simulink library "pmm"  (R2021b)
settings: Solver=VariableStepAuto  StartTime=0.0  StopTime=10.0  RelTol=1e-3
undefined symbols (not defined in the file or in its folder): APMM_CoolgFanActCurr_X_pct, APMM_EWP1Curr_X_c, APMM_EWP3Curr_X_c, APMM_LVBattChktime_X_enum, APMM_LVBattChrgtime_X_enum, APMM_LVChrgLv_X_mV, ENUM_ANTITHEFT_ALARM, ENUM_ANTITHEFT_ARM, ENUM_ANTITHEFT_DISARM, ENUM_ANTITHEFT_WAIT, ENUM_APSSYSTEMSTA_REMOTEACTIVE, ENUM_CHRGPLUGSTA_NONE, ENUM_CRASHSTATE_FRONTFIRSTLV, ENUM_CRASHSTATE_LEFTSIDE, ENUM_CRASHSTATE_RIGHTSIDE, ENUM_DRIVETRAIN_AWD, ENUM_DRIVETRAIN_FWD, ENUM_DRIVETRAIN_RWD, ENUM_GEARACTUALPOSN_D, ENUM_GEARACTUALPOSN_N, ENUM_GEARACTUALPOSN_R, ENUM_HVBATTREADYPRE_READY, ENUM_OTACHKSTA_NOREQUEST, ENUM_OTACHKSTA_NOTIMEOUT, ENUM_OTACHKSTA_TIMEOUT, ENUM_PDKEYRAWLULOCK_INLOCK, ENUM_PDKEYRAWLULOCK_INUNLOCK, ENUM_PDKEYRAWPS_INPS, ENUM_PDKEYSTA_LOCK, ENUM_PDKEYSTA_PS, ENUM_PDKEYSTA_UNAVALIABLE, ENUM_PDKEYSTA_UNLOCK, ENUM_POWERSTA_OFF, ENUM_POWERSTA_OFFC, ENUM_POWERSTA_STANDBY, ENUM_PWRREQOTA_NOREQUEST, ENUM_PWRREQOTA_REQPOWEROFF, ENUM_PWRREQOTA_REQPOWERSTDBY, ENUM_PWRSTASW_READY, ENUM_V2LSTA_NOPLUG, ENUM_VEHICLETYPE_D31L24, FALSE, KPMM_AllDoorClosedHoldTime_s, KPMM_APSAllowThd_pct, KPMM_BattDownFailtime_s, KPMM_BattUpFailtime_s, KPMM_BattUpResetRty_cnt, KPMM_BattUpResetSW_flg, KPMM_BattUpResetTO_s, KPMM_BattUpRstDlyTO_s, KPMM_BrakeSWHoldTime_s, KPMM_ChrgPlugHoldTime_s, KPMM_DCDCDisableFailtime_s, KPMM_DCDCEnableFailtime_s, KPMM_DCDCVSET_V, KPMM_DCDCVSETLVChrg_V, KPMM_DoorSWHoldTime_s, KPMM_DriverSafetyChkFailtime_s, KPMM_DrivetrainSelect_enum_ovrdflg, KPMM_DrivetrainSelect_enum_ovrdval ... (+61)
libraries: simulink x29, hcu_lib x17
(part 3 of 6)

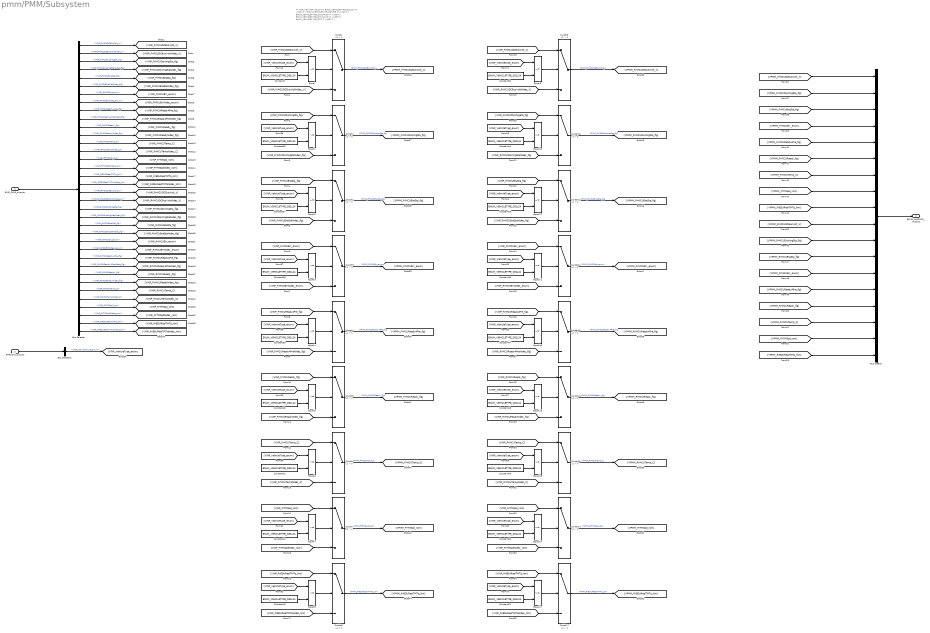
== system pmm/PMM/Subsystem ==
  note: % VINP_VehicleType_enum
      | ENUM_VEHICLETYPE_D31L24         	= uint8(  0  );
      | ENUM_VEHICLETYPE_D31F25         	= uint8(  1  );
      | ENUM_VEHICLETYPE_D31HRWD        = uint8(  2  );
      | ENUM_VEHICLETYPE_D31HAWD        = uint8(  3  );
      | ENUM_VEHICLETYPE_D21           		= uint8(  4  );
  BINP_CAN3_outputs : Inport
  BINP_SYS_outputs : Inport  Port=2
  Bus Creator : BusCreator  Inputs=18
  Bus Selector : BusSelector  OutputSignals=VINP_FrMCUDCBusVolt_V,VINP_FrMCUDCBusVoltNidec_V,VINP_FrMCUDischrgSta_flg,VINP_FrMCUDischrgStaNidec_flg,VINP_FrMCUEnaSta_flg,VINP_FrMCUEnaStaNidec_flg,VINP_FrMCUErr_enum,VINP_FrMCUErrNidec_enum,VINP_FrMCUReady4Pre_flg,VINP_FrMCUReady4PreNidec_flg,VINP_FrMCUReady_flg,VINP_FrMCUReadyNidec_flg,VINP_FrMCUTemp_C,VINP_FrMCUTempNidec_C,VINP_FrTMSpd_rpm,VINP_FrTMSpdNidec_rpm,VINP_FrEDURealTMTq_Nm,VINP_FrEDURealTMTqNidec_Nm,VINP_RrMCUDCBusVolt_V,VINP_RrMCUDCBusVoltNidec_V,VINP_RrMCUDischrgSta_flg,VINP_RrMCUDischrgStaNidec_flg,VINP_RrMCUEnaSta_flg,VINP_RrMCUEnaStaNidec_flg,VINP_RrMCUErr_enum,VINP_RrMCUErrNidec_enum,VINP_RrMCUReady4Pre_flg,VINP_RrMCUReady4PreNidec_flg,VINP_RrMCUReady_flg,VINP_RrMCUReadyNidec_flg,VINP_RrMCUTemp_C,VINP_RrMCUTempNidec_C,VINP_RrTMSpd_rpm,VINP_RrTMSpdNidec_rpm,VINP_RrEDURealTMTq_Nm,VINP_RrEDURealTMTqNidec_Nm
  Bus Selector1 : BusSelector  OutputSignals=VINP_VehicleType_enum
  Constant{1,36..52} (18 alike) : Constant  Value=ENUM_VEHICLETYPE_D31L24
  Equal{,1..17} (18 alike) : RelationalOperator  Operator=~=  OutDataTypeStr=boolean  RndMeth=Simplest
  Switch{,1..17} (18 alike) : Switch  Criteria=u2 > Threshold
  BPMM_CAN3MCU_outputs : Outport
  wires:
  BINP_CAN3_outputs/1 -> Bus Selector/1
  Bus Selector/1 -> [VINP_FrMCUDCBusVolt_V]  "<VINP_FrMCUDCBusVolt_V>"
  Bus Selector/2 -> [VINP_FrMCUDCBusVoltNidec_V]  "<VINP_FrMCUDCBusVoltNidec_V>"
  Bus Selector/3 -> [VINP_FrMCUDischrgSta_flg]  "<VINP_FrMCUDischrgSta_flg>"
  Bus Selector/4 -> [VINP_FrMCUDischrgStaNidec_flg]  "<VINP_FrMCUDischrgStaNidec_flg>"
  Bus Selector/5 -> [VINP_FrMCUEnaSta_flg]  "<VINP_FrMCUEnaSta_flg>"
  Bus Selector/6 -> [VINP_FrMCUEnaStaNidec_flg]  "<VINP_FrMCUEnaStaNidec_flg>"
  Bus Selector/7 -> [VINP_FrMCUErr_enum]  "<VINP_FrMCUErr_enum>"
  Bus Selector/8 -> [VINP_FrMCUErrNidec_enum]  "<VINP_FrMCUErrNidec_enum>"
  Bus Selector/9 -> [VINP_FrMCUReady4Pre_flg]  "<VINP_FrMCUReady4Pre_flg>"
  Bus Selector/10 -> [VINP_FrMCUReady4PreNidec_flg]  "<VINP_FrMCUReady4PreNidec_flg>"
  Bus Selector/11 -> [VINP_FrMCUReady_flg]  "<VINP_FrMCUReady_flg>"
  Bus Selector/12 -> [VINP_FrMCUReadyNidec_flg]  "<VINP_FrMCUReadyNidec_flg>"
  Bus Selector/13 -> [VINP_FrMCUTemp_C]  "<VINP_FrMCUTemp_C>"
  Bus Selector/14 -> [VINP_FrMCUTempNidec_C]  "<VINP_FrMCUTempNidec_C>"
  Bus Selector/15 -> [VINP_FrTMSpd_rpm]  "<VINP_FrTMSpd_rpm>"
  Bus Selector/16 -> [VINP_FrTMSpdNidec_rpm]  "<VINP_FrTMSpdNidec_rpm>"
  Bus Selector/17 -> [VINP_FrEDURealTMTq_Nm]  "<VINP_FrEDURealTMTq_Nm>"
  Bus Selector/18 -> [VINP_FrEDURealTMTqNidec_Nm]  "<VINP_FrEDURealTMTqNidec_Nm>"
  Bus Selector/19 -> [VINP_RrMCUDCBusVolt_V]  "<VINP_RrMCUDCBusVolt_V>"
  Bus Selector/20 -> [VINP_RrMCUDCBusVoltNidec_V]  "<VINP_RrMCUDCBusVoltNidec_V>"
  Bus Selector/21 -> [VINP_RrMCUDischrgSta_flg]  "<VINP_RrMCUDischrgSta_flg>"
  Bus Selector/22 -> [VINP_RrMCUDischrgStaNidec_flg]  "<VINP_RrMCUDischrgStaNidec_flg>"
  Bus Selector/23 -> [VINP_RrMCUEnaSta_flg]  "<VINP_RrMCUEnaSta_flg>"
  Bus Selector/24 -> [VINP_RrMCUEnaStaNidec_flg]  "<VINP_RrMCUEnaStaNidec_flg>"
  Bus Selector/25 -> [VINP_RrMCUErr_enum]  "<VINP_RrMCUErr_enum>"
  Bus Selector/26 -> [VINP_RrMCUErrNidec_enum]  "<VINP_RrMCUErrNidec_enum>"
  Bus Selector/27 -> [VINP_RrMCUReady4Pre_flg]  "<VINP_RrMCUReady4Pre_flg>"
  Bus Selector/28 -> [VINP_RrMCUReady4PreNidec_flg]  "<VINP_RrMCUReady4PreNidec_flg>"
  Bus Selector/29 -> [VINP_RrMCUReady_flg]  "<VINP_RrMCUReady_flg>"
  Bus Selector/30 -> [VINP_RrMCUReadyNidec_flg]  "<VINP_RrMCUReadyNidec_flg>"
  Bus Selector/31 -> [VINP_RrMCUTemp_C]  "<VINP_RrMCUTemp_C>"
  Bus Selector/32 -> [VINP_RrMCUTempNidec_C]  "<VINP_RrMCUTempNidec_C>"
  Bus Selector/33 -> [VINP_RrTMSpd_rpm]  "<VINP_RrTMSpd_rpm>"
  Bus Selector/34 -> [VINP_RrTMSpdNidec_rpm]  "<VINP_RrTMSpdNidec_rpm>"
  Bus Selector/35 -> [VINP_RrEDURealTMTq_Nm]  "<VINP_RrEDURealTMTq_Nm>"
  Bus Selector/36 -> [VINP_RrEDURealTMTqNidec_Nm]  "<VINP_RrEDURealTMTqNidec_Nm>"
  Constant1/1 -> Equal/2
  Equal/1 -> Switch/2
  [VINP_FrMCUDCBusVolt_V] -> Switch/1
  [VINP_FrMCUDCBusVoltNidec_V] -> Switch/3
  Switch/1 -> [VPMM_FrMCUDCBusVolt_V]  "VPMM_FrMCUDCBusVolt_V"
  Equal1/1 -> Switch1/2
  Equal2/1 -> Switch2/2
  [VINP_FrMCUEnaStaNidec_flg] -> Switch2/3
  [VINP_FrMCUEnaSta_flg] -> Switch2/1
  [VINP_FrMCUDischrgStaNidec_flg] -> Switch1/3
  [VINP_FrMCUDischrgSta_flg] -> Switch1/1
  Equal3/1 -> Switch3/2
  [VINP_FrMCUErr_enum] -> Switch3/1
  [VINP_FrMCUErrNidec_enum] -> Switch3/3
  Equal4/1 -> Switch4/2
  [VINP_FrMCUReady4Pre_flg] -> Switch4/1
  [VINP_FrMCUReady4PreNidec_flg] -> Switch4/3
  Equal5/1 -> Switch5/2
  [VINP_FrMCUReady_flg] -> Switch5/1
  [VINP_FrMCUReadyNidec_flg] -> Switch5/3
  Equal6/1 -> Switch6/2
  [VINP_FrMCUTemp_C] -> Switch6/1
  [VINP_FrMCUTempNidec_C] -> Switch6/3
  Equal7/1 -> Switch7/2
  Equal8/1 -> Switch8/2
  [VINP_FrTMSpd_rpm] -> Switch7/1
  [VINP_FrTMSpdNidec_rpm] -> Switch7/3
  [VINP_FrEDURealTMTq_Nm] -> Switch8/1
  [VINP_FrEDURealTMTqNidec_Nm] -> Switch8/3
  Equal9/1 -> Switch9/2
  Equal10/1 -> Switch10/2
  Equal11/1 -> Switch11/2
  Equal12/1 -> Switch12/2
  Equal15/1 -> Switch15/2
  Equal14/1 -> Switch14/2
  Equal13/1 -> Switch13/2
  Equal16/1 -> Switch16/2
  Equal17/1 -> Switch17/2
  [VINP_RrMCUDCBusVolt_V] -> Switch9/1
  [VINP_RrMCUDCBusVoltNidec_V] -> Switch9/3
  [VINP_RrMCUDischrgSta_flg] -> Switch10/1
  [VINP_RrMCUDischrgStaNidec_flg] -> Switch10/3
  [VINP_RrMCUEnaSta_flg] -> Switch12/1
  [VINP_RrMCUEnaStaNidec_flg] -> Switch12/3
  [VINP_RrMCUErr_enum] -> Switch11/1
  [VINP_RrMCUErrNidec_enum] -> Switch11/3
  [VINP_RrMCUReady4Pre_flg] -> Switch16/1
  [VINP_RrMCUReady4PreNidec_flg] -> Switch16/3
  [VINP_RrMCUReady_flg] -> Switch13/1
  [VINP_RrMCUReadyNidec_flg] -> Switch13/3
  [VINP_RrMCUTemp_C] -> Switch15/1
  [VINP_RrMCUTempNidec_C] -> Switch15/3
  [VINP_RrTMSpd_rpm] -> Switch14/1
  [VINP_RrTMSpdNidec_rpm] -> Switch14/3
  [VINP_RrEDURealTMTqNidec_Nm] -> Switch17/3
  [VINP_RrEDURealTMTq_Nm] -> Switch17/1
  Switch1/1 -> [VPMM_FrMCUDischrgSta_flg]  "VPMM_FrMCUDischrgSta_flg"
  Switch2/1 -> [VPMM_FrMCUEnaSta_flg]  "VPMM_FrMCUEnaSta_flg"
  Switch3/1 -> [VPMM_FrMCUErr_enum]  "VPMM_FrMCUErr_enum"
  Switch4/1 -> [VPMM_FrMCUReady4Pre_flg]  "VPMM_FrMCUReady4Pre_flg"
  Switch5/1 -> [VPMM_FrMCUReady_flg]  "VPMM_FrMCUReady_flg"
  Switch6/1 -> [VPMM_FrMCUTemp_C]  "VPMM_FrMCUTemp_C"
  Switch7/1 -> [VPMM_FrTMSpd_rpm]  "VPMM_FrTMSpd_rpm"
  Switch8/1 -> [VPMM_FrEDURealTMTq_Nm]  "VPMM_FrEDURealTMTq_Nm"
  Switch9/1 -> [VPMM_RrMCUDCBusVolt_V]  "VPMM_RrMCUDCBusVolt_V"
  Switch10/1 -> [VPMM_RrMCUDischrgSta_flg]  "VPMM_RrMCUDischrgSta_flg"
  Switch12/1 -> [VPMM_RrMCUEnaSta_flg]  "VPMM_RrMCUEnaSta_flg"
  Switch11/1 -> [VPMM_RrMCUErr_enum]  "VPMM_RrMCUErr_enum"
  Switch16/1 -> [VPMM_RrMCUReady4Pre_flg]  "VPMM_RrMCUReady4Pre_flg"
  Switch13/1 -> [VPMM_RrMCUReady_flg]  "VPMM_RrMCUReady_flg"
  Switch15/1 -> [VPMM_RrMCUTemp_C]  "VPMM_RrMCUTemp_C"
  Switch14/1 -> [VPMM_RrTMSpd_rpm]  "VPMM_RrTMSpd_rpm"
  Switch17/1 -> [VPMM_RrEDURealTMTq_Nm]  "VPMM_RrEDURealTMTq_Nm"
  [VPMM_FrMCUReady_flg] -> Bus Creator/6
  [VPMM_FrMCUReady4Pre_flg] -> Bus Creator/5
  [VPMM_FrMCUTemp_C] -> Bus Creator/7
  [VPMM_FrMCUErr_enum] -> Bus Creator/4
  [VPMM_FrTMSpd_rpm] -> Bus Creator/8
  [VPMM_FrMCUEnaSta_flg] -> Bus Creator/3
  [VPMM_FrEDURealTMTq_Nm] -> Bus Creator/9
  [VPMM_FrMCUDischrgSta_flg] -> Bus Creator/2
  [VPMM_RrMCUDischrgSta_flg] -> Bus Creator/11
  [VPMM_RrMCUEnaSta_flg] -> Bus Creator/12
  [VPMM_RrMCUErr_enum] -> Bus Creator/13
  [VPMM_RrMCUReady4Pre_flg] -> Bus Creator/14
  [VPMM_RrMCUReady_flg] -> Bus Creator/15
  [VPMM_RrMCUTemp_C] -> Bus Creator/16
  [VPMM_RrTMSpd_rpm] -> Bus Creator/17
  [VPMM_RrEDURealTMTq_Nm] -> Bus Creator/18
  Bus Creator/1 -> BPMM_CAN3MCU_outputs/1
  [VPMM_FrMCUDCBusVolt_V] -> Bus Creator/1
  [VPMM_RrMCUDCBusVolt_V] -> Bus Creator/10
  BINP_SYS_outputs/1 -> Bus Selector1/1
  Bus Selector1/1 -> [VINP_VehicleType_enum]  "<VINP_VehicleType_enum>"
  [VINP_VehicleType_enum] -> Equal/1
  [VINP_VehicleType_enum] -> Equal1/1
  Constant36/1 -> Equal1/2
  [VINP_VehicleType_enum] -> Equal2/1
  Constant37/1 -> Equal2/2
  [VINP_VehicleType_enum] -> Equal3/1
  Constant38/1 -> Equal3/2
  [VINP_VehicleType_enum] -> Equal4/1
  Constant39/1 -> Equal4/2
  [VINP_VehicleType_enum] -> Equal5/1
  Constant40/1 -> Equal5/2
  [VINP_VehicleType_enum] -> Equal6/1
  Constant41/1 -> Equal6/2
  [VINP_VehicleType_enum] -> Equal7/1
  Constant42/1 -> Equal7/2
  [VINP_VehicleType_enum] -> Equal8/1
  Constant43/1 -> Equal8/2
  [VINP_VehicleType_enum] -> Equal9/1
  Constant52/1 -> Equal9/2
  [VINP_VehicleType_enum] -> Equal10/1
  Constant44/1 -> Equal10/2
  [VINP_VehicleType_enum] -> Equal12/1
  Constant45/1 -> Equal12/2
  [VINP_VehicleType_enum] -> Equal11/1
  Constant46/1 -> Equal11/2
  [VINP_VehicleType_enum] -> Equal16/1
  Constant47/1 -> Equal16/2
  [VINP_VehicleType_enum] -> Equal13/1
  Constant48/1 -> Equal13/2
  [VINP_VehicleType_enum] -> Equal15/1
  Constant49/1 -> Equal15/2
  [VINP_VehicleType_enum] -> Equal14/1
  Constant50/1 -> Equal14/2
  [VINP_VehicleType_enum] -> Equal17/1
  Constant51/1 -> Equal17/2

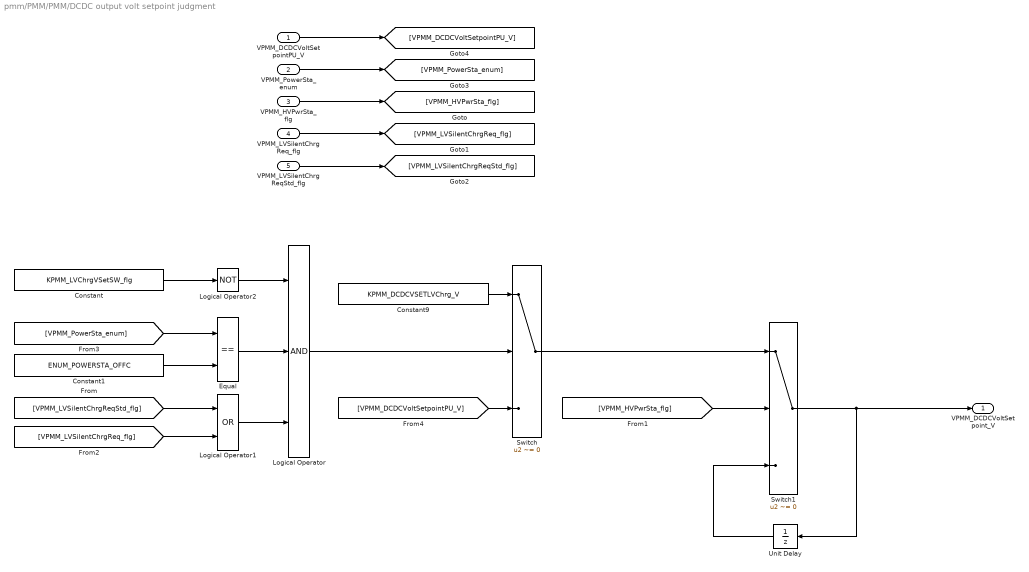
== system pmm/PMM/PMM/DCDC output volt setpoint judgment ==
  VPMM_DCDCVoltSetpointPU_V : Inport
  VPMM_PowerSta_enum : Inport  Port=2
  VPMM_HVPwrSta_flg : Inport  Port=3
  VPMM_LVSilentChrgReq_flg : Inport  Port=4
  VPMM_LVSilentChrgReqStd_flg : Inport  Port=5
  Constant : Constant  Value=KPMM_LVChrgVSetSW_flg
  Constant1 : Constant  Value=ENUM_POWERSTA_OFFC
  Constant9 : Constant  Value=KPMM_DCDCVSETLVChrg_V
  Equal : RelationalOperator  Operator===  OutDataTypeStr=boolean  RndMeth=Simplest
  Logical Operator : Logic  Inputs=3  AllPortsSameDT=off  OutDataTypeStr=boolean
  Logical Operator1 : Logic  Operator=OR  AllPortsSameDT=off  OutDataTypeStr=boolean
  Logical Operator2 : Logic  Operator=NOT  AllPortsSameDT=off  OutDataTypeStr=boolean
  Switch : Switch  Criteria=u2 ~= 0
  Switch1 : Switch  Criteria=u2 ~= 0
  Unit Delay : UnitDelay  SampleTime=-1  HasFrameUpgradeWarning=on
  VPMM_DCDCVoltSetpoint_V : Outport
  wires:
  Switch1/1 -> VPMM_DCDCVoltSetpoint_V/1, Unit Delay/1
  VPMM_PowerSta_enum/1 -> [VPMM_PowerSta_enum]
  VPMM_HVPwrSta_flg/1 -> [VPMM_HVPwrSta_flg]
  VPMM_LVSilentChrgReq_flg/1 -> [VPMM_LVSilentChrgReq_flg]
  VPMM_LVSilentChrgReqStd_flg/1 -> [VPMM_LVSilentChrgReqStd_flg]
  VPMM_DCDCVoltSetpointPU_V/1 -> [VPMM_DCDCVoltSetpointPU_V]
  Constant9/1 -> Switch/1
  Equal/1 -> Logical Operator/2
  Unit Delay/1 -> Switch1/3
  Switch/1 -> Switch1/1
  Logical Operator/1 -> Switch/2
  [VPMM_LVSilentChrgReq_flg] -> Logical Operator1/2
  [VPMM_LVSilentChrgReqStd_flg] -> Logical Operator1/1
  Logical Operator1/1 -> Logical Operator/3
  [VPMM_HVPwrSta_flg] -> Switch1/2
  Constant1/1 -> Equal/2
  [VPMM_PowerSta_enum] -> Equal/1
  [VPMM_DCDCVoltSetpointPU_V] -> Switch/3
  Logical Operator2/1 -> Logical Operator/1
  Constant/1 -> Logical Operator2/1

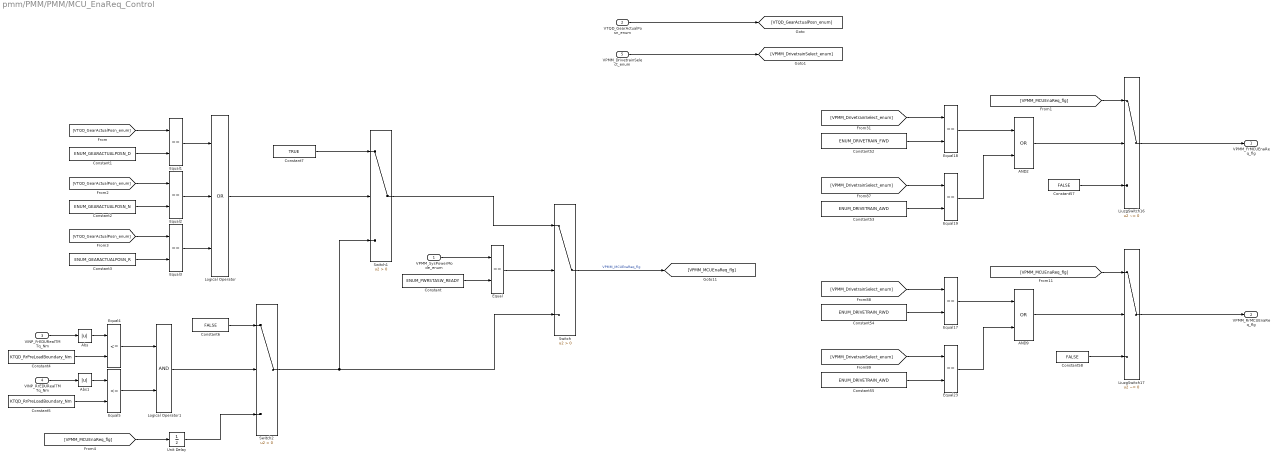
== system pmm/PMM/PMM/MCU_EnaReq_Control ==
  VPMM_SysPowerMode_enum : Inport
  VTQD_GearActualPosn_enum : Inport  Port=2
  VINP_FrEDURealTMTq_Nm : Inport  Port=3
  VINP_RrEDURealTMTq_Nm : Inport  Port=4
  VPMM_DrivetrainSelect_enum : Inport  Port=5
  AND2 : Logic  Operator=OR  AllPortsSameDT=off  OutDataTypeStr=boolean
  AND9 : Logic  Operator=OR  AllPortsSameDT=off  OutDataTypeStr=boolean
  Abs : Abs
  Abs1 : Abs
  Constant : Constant  Value=ENUM_PWRSTASW_READY
  Constant1 : Constant  Value=ENUM_GEARACTUALPOSN_D
  Constant2 : Constant  Value=ENUM_GEARACTUALPOSN_N
  Constant3 : Constant  Value=ENUM_GEARACTUALPOSN_R
  Constant4 : Constant  Value=KTQD_RrPreLoadBoundary_Nm
  Constant5 : Constant  Value=KTQD_RrPreLoadBoundary_Nm
  Constant52 : Constant  Value=ENUM_DRIVETRAIN_FWD
  Constant53 : Constant  Value=ENUM_DRIVETRAIN_AWD
  Constant54 : Constant  Value=ENUM_DRIVETRAIN_RWD
  Constant55 : Constant  Value=ENUM_DRIVETRAIN_AWD
  Constant57 : Constant  Value=FALSE
  Constant58 : Constant  Value=FALSE
  Constant6 : Constant  Value=FALSE
  Constant7 : Constant  Value=TRUE
  Equal{,1..3,17..19,23} (8 alike) : RelationalOperator  Operator===  OutDataTypeStr=boolean  RndMeth=Simplest
  Equal4 : RelationalOperator  Operator=<=  OutDataTypeStr=boolean  RndMeth=Simplest
  Equal5 : RelationalOperator  Operator=<=  OutDataTypeStr=boolean  RndMeth=Simplest
  LiuzgSwitch16 : Switch  Criteria=u2 ~= 0
      settings: AttributesFormatString=<%<Criteria>>
  LiuzgSwitch17 : Switch  Criteria=u2 ~= 0
      settings: AttributesFormatString=<%<Criteria>>
  Logical Operator : Logic  Operator=OR  Inputs=3  AllPortsSameDT=off  OutDataTypeStr=boolean
  Logical Operator1 : Logic  AllPortsSameDT=off  OutDataTypeStr=boolean
  Switch : Switch  Criteria=u2 > Threshold
  Switch1 : Switch  Criteria=u2 > Threshold
  Switch2 : Switch  Criteria=u2 > Threshold
  Unit Delay : UnitDelay  SampleTime=-1  HasFrameUpgradeWarning=on
  VPMM_FrMCUEnaReq_flg : Outport
  VPMM_RrMCUEnaReq_flg : Outport  Port=2
  wires:
  VPMM_DrivetrainSelect_enum/1 -> [VPMM_DrivetrainSelect_enum]
  LiuzgSwitch17/1 -> VPMM_RrMCUEnaReq_flg/1
  Constant57/1 -> LiuzgSwitch16/3
  [VPMM_DrivetrainSelect_enum] -> Equal19/1
  Constant55/1 -> Equal23/2
  Constant58/1 -> LiuzgSwitch17/3
  Constant54/1 -> Equal17/2
  Constant53/1 -> Equal19/2
  Equal19/1 -> AND2/2
  [VPMM_DrivetrainSelect_enum] -> Equal17/1
  [VPMM_MCUEnaReq_flg] -> LiuzgSwitch16/1
  [VPMM_MCUEnaReq_flg] -> LiuzgSwitch17/1
  AND2/1 -> LiuzgSwitch16/2
  [VPMM_DrivetrainSelect_enum] -> Equal23/1
  Equal17/1 -> AND9/1
  Constant52/1 -> Equal18/2
  [VPMM_DrivetrainSelect_enum] -> Equal18/1
  Equal18/1 -> AND2/1
  LiuzgSwitch16/1 -> VPMM_FrMCUEnaReq_flg/1
  AND9/1 -> LiuzgSwitch17/2
  Equal23/1 -> AND9/2
  VPMM_SysPowerMode_enum/1 -> Equal/1
  Constant/1 -> Equal/2
  Equal/1 -> Switch/2
  Switch1/1 -> Switch/1
  Switch/1 -> [VPMM_MCUEnaReq_flg]  "VPMM_MCUEnaReq_flg"
  VTQD_GearActualPosn_enum/1 -> [VTQD_GearActualPosn_enum]
  [VTQD_GearActualPosn_enum] -> Equal1/1
  [VTQD_GearActualPosn_enum] -> Equal2/1
  [VTQD_GearActualPosn_enum] -> Equal3/1
  Constant3/1 -> Equal3/2
  Constant2/1 -> Equal2/2
  Constant1/1 -> Equal1/2
  Equal3/1 -> Logical Operator/3
  Equal2/1 -> Logical Operator/2
  Equal1/1 -> Logical Operator/1
  Logical Operator/1 -> Switch1/2
  Switch2/1 -> Switch1/3, Switch/3
  Equal4/1 -> Logical Operator1/1
  Equal5/1 -> Logical Operator1/2
  Logical Operator1/1 -> Switch2/2
  VINP_FrEDURealTMTq_Nm/1 -> Abs/1
  VINP_RrEDURealTMTq_Nm/1 -> Abs1/1
  Constant4/1 -> Equal4/2
  Constant5/1 -> Equal5/2
  [VPMM_MCUEnaReq_flg] -> Unit Delay/1
  Unit Delay/1 -> Switch2/3
  Constant6/1 -> Switch2/1
  Constant7/1 -> Switch1/1
  Abs/1 -> Equal4/1
  Abs1/1 -> Equal5/1

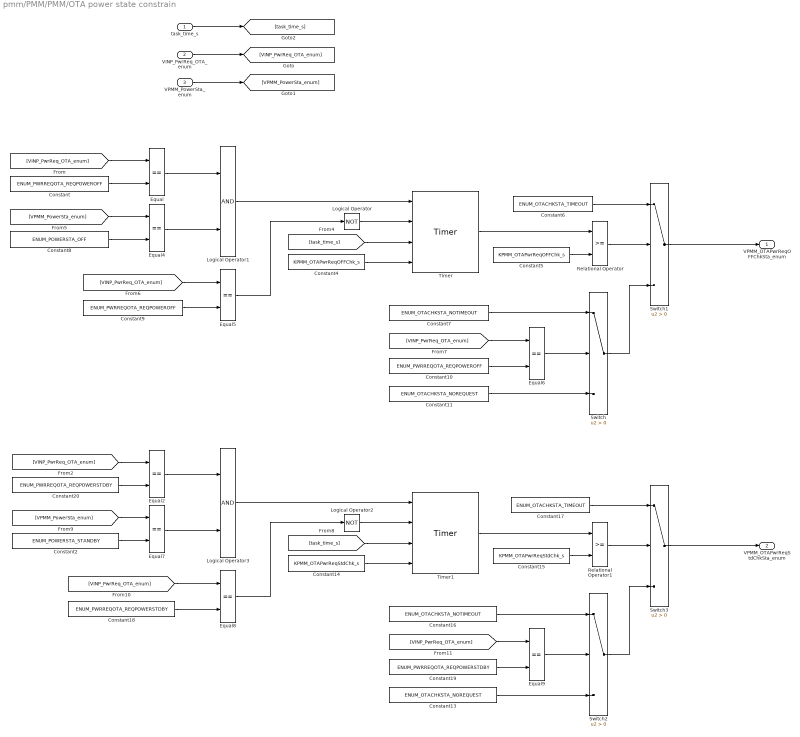
== system pmm/PMM/PMM/OTA power state constrain ==
  task_time_s : Inport
  VINP_PwrReq_OTA_enum : Inport  Port=2
  VPMM_PowerSta_enum : Inport  Port=3
  Constant : Constant  Value=ENUM_PWRREQOTA_REQPOWEROFF
  Constant10 : Constant  Value=ENUM_PWRREQOTA_REQPOWEROFF
  Constant11 : Constant  Value=ENUM_OTACHKSTA_NOREQUEST
  Constant13 : Constant  Value=ENUM_OTACHKSTA_NOREQUEST
  Constant14 : Constant  Value=KPMM_OTAPwrReqStdChk_s
  Constant15 : Constant  Value=KPMM_OTAPwrReqStdChk_s
  Constant16 : Constant  Value=ENUM_OTACHKSTA_NOTIMEOUT
  Constant17 : Constant  Value=ENUM_OTACHKSTA_TIMEOUT
  Constant18 : Constant  Value=ENUM_PWRREQOTA_REQPOWERSTDBY
  Constant19 : Constant  Value=ENUM_PWRREQOTA_REQPOWERSTDBY
  Constant2 : Constant  Value=ENUM_POWERSTA_STANDBY
  Constant20 : Constant  Value=ENUM_PWRREQOTA_REQPOWERSTDBY
  Constant4 : Constant  Value=KPMM_OTAPwrReqOFFChk_s
  Constant5 : Constant  Value=KPMM_OTAPwrReqOFFChk_s
  Constant6 : Constant  Value=ENUM_OTACHKSTA_TIMEOUT
  Constant7 : Constant  Value=ENUM_OTACHKSTA_NOTIMEOUT
  Constant8 : Constant  Value=ENUM_POWERSTA_OFF
  Constant9 : Constant  Value=ENUM_PWRREQOTA_REQPOWEROFF
  Equal{,2,4..9} (8 alike) : RelationalOperator  Operator===  OutDataTypeStr=boolean  RndMeth=Simplest
  Logical Operator : Logic  Operator=NOT  AllPortsSameDT=off  OutDataTypeStr=boolean
  Logical Operator1 : Logic  AllPortsSameDT=off  OutDataTypeStr=boolean
  Logical Operator2 : Logic  Operator=NOT  AllPortsSameDT=off  OutDataTypeStr=boolean
  Logical Operator3 : Logic  AllPortsSameDT=off  OutDataTypeStr=boolean
  Relational Operator : RelationalOperator  OutDataTypeStr=boolean  RndMeth=Simplest
  Relational Operator1 : RelationalOperator  OutDataTypeStr=boolean  RndMeth=Simplest
  Switch{,1..3} (4 alike) : Switch  Criteria=u2 > Threshold
  Timer : hcu_lib/Basic_Blocks/Timer
  Timer1 : hcu_lib/Basic_Blocks/Timer
  VPMM_OTAPwrReqOFFChkSta_enum : Outport
  VPMM_OTAPwrReqStdChkSta_enum : Outport  Port=2
  wires:
  Constant/1 -> Equal/2
  VINP_PwrReq_OTA_enum/1 -> [VINP_PwrReq_OTA_enum]
  VPMM_PowerSta_enum/1 -> [VPMM_PowerSta_enum]
  [VINP_PwrReq_OTA_enum] -> Equal/1
  task_time_s/1 -> [task_time_s]
  [task_time_s] -> Timer/3
  Constant4/1 -> Timer/4
  Constant5/1 -> Relational Operator/2
  Timer/1 -> Relational Operator/1
  Relational Operator/1 -> Switch1/2
  Logical Operator/1 -> Timer/2
  Constant8/1 -> Equal4/2
  [VPMM_PowerSta_enum] -> Equal4/1
  Equal/1 -> Logical Operator1/1
  Equal4/1 -> Logical Operator1/2
  Logical Operator1/1 -> Timer/1
  [VINP_PwrReq_OTA_enum] -> Equal5/1
  Constant9/1 -> Equal5/2
  Equal5/1 -> Logical Operator/1
  Constant6/1 -> Switch1/1
  Constant10/1 -> Equal6/2
  [VINP_PwrReq_OTA_enum] -> Equal6/1
  Equal6/1 -> Switch/2
  Constant7/1 -> Switch/1
  Switch/1 -> Switch1/3
  Constant11/1 -> Switch/3
  Switch1/1 -> VPMM_OTAPwrReqOFFChkSta_enum/1
  Switch2/1 -> Switch3/3
  Equal9/1 -> Switch2/2
  [VINP_PwrReq_OTA_enum] -> Equal9/1
  Equal8/1 -> Logical Operator2/1
  [VINP_PwrReq_OTA_enum] -> Equal8/1
  Logical Operator3/1 -> Timer1/1
  Equal7/1 -> Logical Operator3/2
  Equal2/1 -> Logical Operator3/1
  [VPMM_PowerSta_enum] -> Equal7/1
  Logical Operator2/1 -> Timer1/2
  Relational Operator1/1 -> Switch3/2
  Timer1/1 -> Relational Operator1/1
  Constant15/1 -> Relational Operator1/2
  Constant14/1 -> Timer1/4
  [task_time_s] -> Timer1/3
  [VINP_PwrReq_OTA_enum] -> Equal2/1
  Constant20/1 -> Equal2/2
  Constant13/1 -> Switch2/3
  Constant16/1 -> Switch2/1
  Constant17/1 -> Switch3/1
  Switch3/1 -> VPMM_OTAPwrReqStdChkSta_enum/1
  Constant2/1 -> Equal7/2
  Constant18/1 -> Equal8/2
  Constant19/1 -> Equal9/2

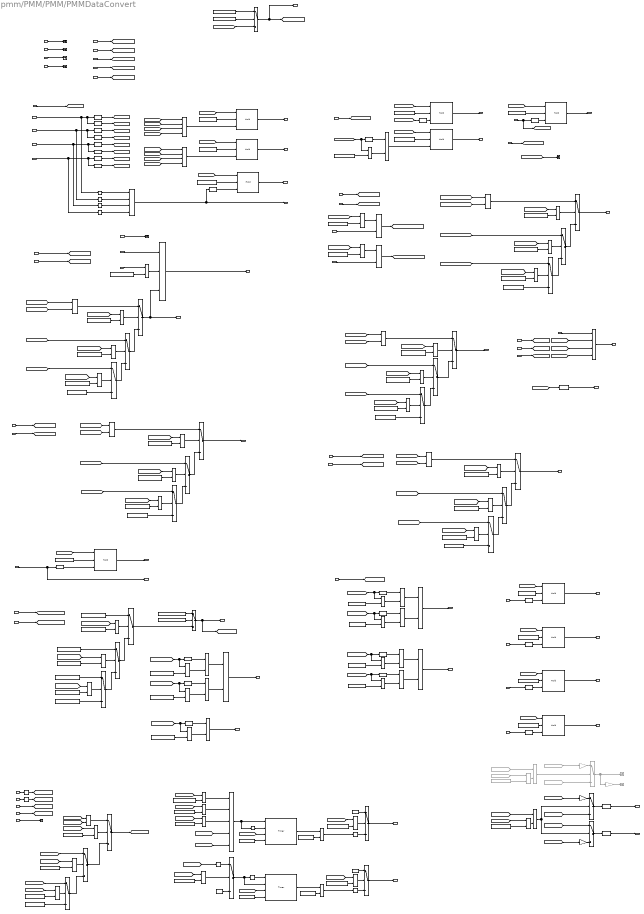
== system pmm/PMM/PMM/PMMDataConvert ==
  note: Comment out to reduce CPU resource.
      | Use below if judgement to avoid float multiply.
  note: Aux Battery Handle
  note: Detect HV power state
  note: Detect PW Continue Use
  note: Detect SchedChgwake
  note: Detect IVI Power OFF
  note: Monitor for DCDC fault level
  note: Safety Check
  note: 0 = HVIL close; 1 = HVIL open
  note: Seat Switch Rising Edge
  note: Detect Gun Plug Rising/Faling Edge
  note: KEY STATE
  note: Brake signal convert to rising edge
  note: Door judgement
  note: Precharge Check
  note: MCU Enable
  note: MCU Discharge
  note: MCU Ready
  note: Antitheft State
  note: OPDS Signal tramsmit function
  note: BMSWarn judgement
  note: MCU DC Bus Max Voltage judgement
  note: VPMM_SafetyChkHLv_flg
      | 0 Fail
      | 1 OK
  note: VPMM_TMSpdThdSta_flg
      | 0 = Not allow MCU disable
      | 1 = Allow MCU disable
  note: 0 = No fail;
      | 1 = fail
  note: VPMM_SafetyChkMLv_flg
      | 0 Fail
      | 1 OK
  task_time_s : Inport
  VBCM_AntitheftSta_enum : Inport  Port=2
  VINP_DrDoorSW_flg : Inport  Port=3
  VINP_PsDoorSW_flg : Inport  Port=4
  VINP_RRDoorSW_flg : Inport  Port=5
  VINP_RLDoorSW_flg : Inport  Port=6
  VINP_BrakeSWGPIO_flg : Inport  Port=7
  VINP_FrMCUDCBusVolt_V : Inport  Port=8
  VINP_FrMCUDischrgSta_flg : Inport  Port=9
  VINP_FrMCUEnaSta_flg : Inport  Port=10
  VINP_FrMCUErr_enum : Inport  Port=11
  VINP_FrMCUReady4Pre_flg : Inport  Port=12
  VINP_FrMCUReady_flg : Inport  Port=13
  VINP_FrMCUTemp_C : Inport  Port=14
  VINP_RrMCUDCBusVolt_V : Inport  Port=15
  VINP_RrMCUDischrgSta_flg : Inport  Port=16
  VINP_RrMCUEnaSta_flg : Inport  Port=17
  VINP_RrMCUErr_enum : Inport  Port=18
  VINP_RrMCUReady4Pre_flg : Inport  Port=19
  VINP_RrMCUReady_flg : Inport  Port=20
  VINP_RrMCUTemp_C : Inport  Port=21
  VINP_DCDCReady4Pre_flg : Inport  Port=22
  VINP_OBCReady4Pre_flg : Inport  Port=23
  VINP_HVBattReady4Pre_enum : Inport  Port=24
  VINP_PDKeyAreaPS_enum : Inport  Port=25
  VINP_PDKeyAreaLockUnlock_enum : Inport  Port=26
  VINP_ChrgPlugSta_enum : Inport  Port=27
  VINP_SeatSW_flg : Inport  Port=28
  VINP_HVILSta_flg : Inport  Port=29
  VINP_CrashOutputSts_enum : Inport  Port=30
  VPMM_PowerSta_enum : Inport  Port=31
  VINP_RrTMSpd_rpm : Inport  Port=32
  VINP_FrTMSpd_rpm : Inport  Port=33
  VINP_BMSWarn5_flg : Inport  Port=34
  VINP_BMSWarn6_flg : Inport  Port=35
  VINP_BMSWarn7_flg : Inport  Port=36
  VINP_BMSWarn8_flg : Inport  Port=37
  VINP_DrivetrainSelect_enum : Inport  Port=38
  VINP_DCDCFaultSta_enum : Inport  Port=39
  VINP_IVIPwroffreq_flg : Inport  Port=40
  VINP_SchedChgwake_flg : Inport  Port=41
  VINP_PWCONTINUEUSE_flg : Inport  Port=42
  VPMM_HVPwrSta_flg : Inport  Port=43
  VINP_LVBattDet12V_V : Inport  Port=44
  VINP_AuxBattVolmV_mV : Inport  Port=45
  VINP_NewNMSpec_flg : Inport  Port=46
  VINP_VehicleType_enum : Inport  Port=47
  AND{,3..6,8} (6 alike) : Logic  AllPortsSameDT=off  OutDataTypeStr=boolean
  AND1 : Logic  Inputs=3  AllPortsSameDT=off  OutDataTypeStr=boolean
  AND7 : Logic  Operator=OR  Inputs=4  AllPortsSameDT=off  OutDataTypeStr=boolean
  Abs : Abs
  Abs1 : Abs
  Constant : Constant  Value=KPMM_DoorSWHoldTime_s
  Constant1 : Constant  Value=KPMM_DoorSWHoldTime_s
  Constant10 : Constant  Commented=on  Value=ENUM_VEHICLETYPE_D31L24
  Constant{4,11,19,22,30,38} (6 alike) : Constant  Value=ENUM_DRIVETRAIN_AWD
  Constant12 : Constant  Value=ENUM_VEHICLETYPE_D31L24
  Constant{6,13,21,32,39,46} (6 alike) : Constant  Value=ENUM_DRIVETRAIN_FWD
  Constant14 : Constant  Value=ENUM_HVBATTREADYPRE_READY
  Constant{8,15,23,34,40,51} (6 alike) : Constant  Value=ENUM_DRIVETRAIN_RWD
  Constant{7,9,16..17,28} (5 alike) : Constant  Value=FALSE
  Constant18 : Constant  Value=KPMM_ChrgPlugHoldTime_s
  Constant2 : Constant  Value=ZERO_FLOAT
  Constant20 : Constant  Value=KPMM_ChrgPlugHoldTime_s
  Constant24 : Constant  Value=KPMM_RrMCUDischrgVolt_V
  Constant25 : Constant  Value=KPMM_FrMCUDischrgVolt_V
  Constant26 : Constant  Value=KPMM_DrivetrainSelect_enum_ovrdflg
  Constant3 : Constant  Value=KPMM_SeatSWHoldTime_s
  Constant31 : Constant  Value=ENUM_CHRGPLUGSTA_NONE
  Constant37 : Constant  Value=KPMM_AllDoorClosedHoldTime_s
  Constant41 : Constant  Value=KPMM_BrakeSWHoldTime_s
  Constant42 : Constant  Value=KPMM_PDKeySta_enum_ovrdval
  Constant43 : Constant  Value=ENUM_PDKEYRAWPS_INPS
  Constant44 : Constant  Value=KPMM_PDKeySta_enum_ovrdflg
  Constant45 : Constant  Value=ENUM_PDKEYRAWLULOCK_INUNLOCK
  Constant47 : Constant  Value=ENUM_PDKEYRAWLULOCK_INLOCK
  Constant48 : Constant  Value=ENUM_PDKEYSTA_UNAVALIABLE
  Constant49 : Constant  Value=ENUM_PDKEYSTA_LOCK
  Constant5 : Constant  Value=ENUM_CRASHSTATE_FRONTFIRSTLV
  Constant50 : Constant  Value=ENUM_PDKEYSTA_UNLOCK
  Constant52 : Constant  Value=KPMM_DrivetrainSelect_enum_ovrdval
  Constant53 : Constant  Value=ENUM_ANTITHEFT_DISARM
  Constant54 : Constant  Value=ENUM_ANTITHEFT_WAIT
  Constant56 : Constant  Value=ENUM_PDKEYSTA_PS
  Constant58 : Constant  Value=ENUM_PDKEYSTA_UNLOCK
  Constant59 : Constant  Value=ENUM_PDKEYSTA_PS
  Constant60 : Constant  Value=ENUM_ANTITHEFT_ARM
  Constant61 : Constant  Value=ENUM_ANTITHEFT_ALARM
  Constant62 : Constant  Value=ENUM_PDKEYSTA_LOCK
  Constant63 : Constant  Value=KPMM_IVIPwroffHoldTime_s
  Constant64 : Constant  Value=KPMM_SchedChgHoldTime_s
  Constant65 : Constant  Value=KPMM_PWCONTINUEHoldTime_s
  Constant66 : Constant  Value=KPMM_HVPwrStaHoldTime_s
  Constant67 : Constant  Value=ENUM_CRASHSTATE_RIGHTSIDE
  Constant68 : Constant  Value=ENUM_CRASHSTATE_LEFTSIDE
  Constant69 : Constant  Value=KPMM_TMSpdMCUDisThrsh_rpm
  Constant70 : Constant  Value=TRUE
  Constant71 : Constant  Value=KPMM_SaftyChkHLvTO_s
  Constant72 : Constant  Value=ENUM_POWERSTA_OFF
  Constant73 : Constant  Value=TRUE
  Constant74 : Constant  Value=KPMM_SaftyChkMLvTO_s
  Constant75 : Constant  Value=KPMM_SaftyChkMLvTO_s
  Constant76 : Constant  Value=TRUE
  Constant77 : Constant  Value=ENUM_POWERSTA_OFF
  Constant79 : Constant  Value=KPMM_SaftyChkHLvTO_s
  Data Type Conversion : DataTypeConversion  OutDataTypeStr=uint8
  Data Type Conversion1 : DataTypeConversion
  Data Type Conversion3 : DataTypeConversion
  Detect Change{,1..6} (7 alike) : simulink/Logic and Bit Operations/Detect Change  vinit=0  OutDataTypeStr=boolean
  Detect Decrease{,1..4} (5 alike) : simulink/Logic and Bit Operations/Detect Decrease  vinit=0.0  OutDataTypeStr=boolean
  Detect Increase{,1..11} (12 alike) : simulink/Logic and Bit Operations/Detect Increase  vinit=0.0  OutDataTypeStr=boolean
  Equal{,1..9,12,14..18,20..22,24..25,27..38,41,44} (35 alike) : RelationalOperator  Operator===  OutDataTypeStr=boolean  RndMeth=Simplest
  Equal10 : RelationalOperator  Operator=<=  OutDataTypeStr=boolean  RndMeth=Simplest
  Equal11 : RelationalOperator  Operator=<=  OutDataTypeStr=boolean  RndMeth=Simplest
  Equal13 : RelationalOperator  Commented=on  Operator=~=  OutDataTypeStr=boolean  RndMeth=Simplest
  Equal26 : RelationalOperator  Operator=~=  OutDataTypeStr=boolean  RndMeth=Simplest
  Equal40 : RelationalOperator  OutDataTypeStr=boolean  RndMeth=Simplest
  Equal42 : RelationalOperator  OutDataTypeStr=boolean  RndMeth=Simplest
  Equal43 : RelationalOperator  Operator=<  OutDataTypeStr=boolean  RndMeth=Simplest
  From93 : From  Commented=on  GotoTag=VINP_VehicleType_enum
  From94 : From  Commented=on  GotoTag=VINP_NewNMSpec_flg
  From95 : From  Commented=on  GotoTag=VINP_AuxBattVolmV_mV
  From96 : From  Commented=on  GotoTag=VINP_LVBattDet12V_V
  Gain : Gain  Commented=on  Gain=1000
  Gain1 : Gain  Commented=on  Gain=0.001
  Gain2 : Gain  Gain=0.001
  Gain3 : Gain  Gain=1000
  Hold{,1..10} (11 alike) : hcu_lib/Basic_Blocks/Hold  SystemSampleTime=-1  VariantActivationTime=update diagram  Latency=0  AutoFrameSizeCalculation=off
      settings: SourceProductName=HCU Relative Block Library
  LiuzgSwitch{1..18,20..27} (26 alike) : Switch  Criteria=u2 ~= 0
      settings: AttributesFormatString=<%<Criteria>>
  LiuzgSwitch19 : Switch  Commented=on  Criteria=u2 ~= 0
      settings: AttributesFormatString=<%<Criteria>>
  Logical Operator{1..3,5..6,8..9,11,14} (9 alike) : Logic  AllPortsSameDT=off  OutDataTypeStr=boolean
  Logical Operator10 : Logic  Operator=OR  AllPortsSameDT=off  OutDataTypeStr=boolean
  Logical Operator12 : Logic  Commented=on  AllPortsSameDT=off  OutDataTypeStr=boolean
  Logical Operator13 : Logic  Operator=OR  Inputs=5  AllPortsSameDT=off  OutDataTypeStr=boolean
  Logical Operator4 : Logic  Operator=OR  AllPortsSameDT=off  OutDataTypeStr=boolean
  Logical Operator7 : Logic  Operator=OR  AllPortsSameDT=off  OutDataTypeStr=boolean
  Max : MinMax  Function=max  Inputs=2
  Max1 : MinMax  Function=max  Inputs=2
  NOT{2..9,11} (9 alike) : Logic  Operator=NOT  AllPortsSameDT=off  OutDataTypeStr=boolean
  OR : Logic  Operator=OR  Inputs=4  AllPortsSameDT=off  OutDataTypeStr=boolean
  OR1 : Logic  Operator=OR  Inputs=4  AllPortsSameDT=off  OutDataTypeStr=boolean
  OR2 : Logic  Inputs=4  AllPortsSameDT=off  OutDataTypeStr=boolean
  Switch : Switch  Criteria=u2 ~= 0
  Switch1 : Switch  Criteria=u2 ~= 0
  Terminator{,1..6} (7 alike) : Terminator
  Timer : hcu_lib/Basic_Blocks/Timer
  Timer1 : hcu_lib/Basic_Blocks/Timer
  VPMM_AuxBatVolt_V_commentout : Terminator  Commented=on
  VPMM_AuxBatVolt_mV_commentout : Terminator  Commented=on
  VPMM_DetectDoorOpened_flg : Outport
  VPMM_DetectDoorClosed_flg : Outport  Port=2
  VPMM_BrkPedalPressed_flg : Outport  Port=3
  VPMM_PreChrgChk_flg : Outport  Port=4
  VPMM_AllDoorClosed_flg : Outport  Port=5
  VPMM_MCUEnable_flg : Outport  Port=6
  VPMM_MCUDischrgFinished_flg : Outport  Port=7
  VPMM_MCUReady_flg : Outport  Port=8
  VPMM_PDKeySta_enum : Outport  Port=9
  VPMM_BrkPedalRisingEdge_flg : Outport  Port=10
  VPMM_AllDoorCloseRisingEdge_flg : Outport  Port=11
  VPMM_DrivetrainSelect_enum : Outport  Port=12
  VPMM_ChrgPlugInRisingEdge_flg : Outport  Port=13
  VPMM_ChrgPlugOutFallingEdge_flg : Outport  Port=14
  VPMM_SeatSWRisingEdge_flg : Outport  Port=15
  VPMM_SafetyChkMLv_flg : Outport  Port=16
  VPMM_SafetyChkHLv_flg : Outport  Port=17
  VPMM_DrSeatSta_enum : Outport  Port=18
  VPMM_BMSWarm_flg : Outport  Port=19
  VPMM_MCUDCBusMaxVolt_V : Outport  Port=20
  VPMM_DetectAntitheftUnlock_flg : Outport  Port=21
  VPMM_DetectPDKeyUnlock_flg : Outport  Port=22
  VPMM_DetectAntitheftLock_flg : Outport  Port=23
  VPMM_DetectPDKeyLock_flg : Outport  Port=24
  VPMM_DetectIVIPwroffreq_flg : Outport  Port=25
  VPMM_DetectSchedChg_flg : Outport  Port=26
  VPMM_DetectPWCONTINUE_flg : Outport  Port=27
  VPMM_DetectHVPwrSta_flg : Outport  Port=28
  VPMM_MCUReady4Pre_flg : Outport  Port=29
  VPMM_AuxBatVolt_mV : Outport  Port=30
  VPMM_AuxBatVolt_V : Outport  Port=31
  wires:
  Data Type Conversion/1 -> VPMM_DrSeatSta_enum/1  "VPMM_DrSeatSta_enum"
  [VPMM_FrMCUDCBusVolt_V] -> Max1/2
  [VPMM_RrMCUDCBusVolt_V] -> Max1/1
  [VPMM_FrMCUDCBusVolt_V] -> LiuzgSwitch18/1
  Max1/1 -> LiuzgSwitch25/1
  Constant7/1 -> LiuzgSwitch26/3
  Constant46/1 -> Equal30/2
  LiuzgSwitch26/1 -> LiuzgSwitch18/3
  Equal12/1 -> LiuzgSwitch25/2
  Constant51/1 -> Equal31/2
  [VPMM_DrivetrainSelect_enum] -> Equal12/1
  Equal30/1 -> LiuzgSwitch18/2
  Constant22/1 -> Equal12/2
  LiuzgSwitch18/1 -> LiuzgSwitch25/3
  [VPMM_DrivetrainSelect_enum] -> Equal30/1
  Equal31/1 -> LiuzgSwitch26/2
  [VPMM_DrivetrainSelect_enum] -> Equal31/1
  [VPMM_RrMCUDCBusVolt_V] -> LiuzgSwitch26/1
  LiuzgSwitch25/1 -> VPMM_MCUDCBusMaxVolt_V/1  "VPMM_MCUDCBusMaxVolt_V"
  [VPMM_FrMCUDCBusVolt_V] -> Equal11/1
  [VPMM_RrMCUDCBusVolt_V] -> Equal10/1
  VINP_BMSWarn5_flg/1 -> AND7/1
  AND7/1 -> VPMM_BMSWarm_flg/1  "VPMM_BMSWarm_flg"
  [VPMM_SeatSW_flg] -> Data Type Conversion/1
  Abs1/1 -> [VINP_FrTMSpdABS_rpm]
  Abs/1 -> [VINP_RrTMSpdABS_rpm]
  LiuzgSwitch23/1 -> [VPMM_TMSpd_rpm]  "VPMM_TMSpd_rpm"
  Constant2/1 -> LiuzgSwitch24/3
  Max/1 -> LiuzgSwitch23/1
  [VINP_FrTMSpdABS_rpm] -> Max/2
  [VINP_RrTMSpdABS_rpm] -> Max/1
  LiuzgSwitch22/1 -> LiuzgSwitch23/3
  LiuzgSwitch24/1 -> LiuzgSwitch22/3
  [VINP_FrTMSpdABS_rpm] -> LiuzgSwitch22/1
  [VINP_RrTMSpdABS_rpm] -> LiuzgSwitch24/1
  [VPMM_DrivetrainSelect_enum] -> Equal27/1
  Constant40/1 -> Equal29/2
  Constant38/1 -> Equal27/2
  Equal29/1 -> LiuzgSwitch24/2
  Equal27/1 -> LiuzgSwitch23/2
  Constant39/1 -> Equal28/2
  [VPMM_DrivetrainSelect_enum] -> Equal29/1
  Equal28/1 -> LiuzgSwitch22/2
  [VPMM_DrivetrainSelect_enum] -> Equal28/1
  VINP_FrTMSpd_rpm/1 -> Abs1/1
  VINP_RrTMSpd_rpm/1 -> Abs/1
  VPMM_PowerSta_enum/1 -> [VPMM_PowerSta_enum]
  [task_time_s] -> Hold4/1
  Hold4/1 -> VPMM_SeatSWRisingEdge_flg/1  "VPMM_SeatSWRisingEdge_flg"
  VINP_SeatSW_flg/1 -> Detect Increase6/1, [VPMM_SeatSW_flg]
  Constant3/1 -> Hold4/2
  Detect Increase6/1 -> Hold4/3
  Constant18/1 -> Hold6/2
  Hold5/1 -> VPMM_ChrgPlugOutFallingEdge_flg/1  "VPMM_ChrgPlugOutFallingEdge_flg"
  Detect Increase7/1 -> Hold6/3
  [VINP_ChrgPlugSta_enum] -> Detect Increase7/1
  [task_time_s] -> Hold5/1
  VINP_ChrgPlugSta_enum/1 -> [VINP_ChrgPlugSta_enum]
  Constant20/1 -> Hold5/2
  [task_time_s] -> Hold6/1
  Logical Operator1/1 -> Hold5/3
  Hold6/1 -> VPMM_ChrgPlugInRisingEdge_flg/1  "VPMM_ChrgPlugInRisingEdge_flg"
  Equal25/1 -> Logical Operator1/2
  [VINP_ChrgPlugSta_enum] -> Detect Decrease4/1, Equal25/1
  Constant31/1 -> Equal25/2
  Detect Decrease4/1 -> Logical Operator1/1
  Equal24/1 -> AND1/2
  Constant14/1 -> Equal24/2
  Switch/1 -> VPMM_DrivetrainSelect_enum/1, [VPMM_DrivetrainSelect_enum]  "VPMM_DrivetrainSelect_enum"
  Detect Increase5/1 -> Hold2/3
  Hold2/1 -> VPMM_AllDoorCloseRisingEdge_flg/1  "VPMM_AllDoorCloseRisingEdge_flg"
  Constant37/1 -> Hold2/2
  [task_time_s] -> Hold2/1
  VINP_OBCReady4Pre_flg/1 -> Terminator1/1
  VINP_HVBattReady4Pre_enum/1 -> Equal24/1
  LiuzgSwitch14/1 -> Switch1/3
  Constant42/1 -> Switch1/1
  Switch1/1 -> [VPMM_PDKeySta_enum], VPMM_PDKeySta_enum/1  "VPMM_PDKeySta_enum"
  Constant44/1 -> Switch1/2
  Constant50/1 -> LiuzgSwitch13/1
  Constant56/1 -> LiuzgSwitch14/1
  Constant49/1 -> LiuzgSwitch15/1
  [VINP_PDKeyAreaLockUnlock_enum] -> Equal22/1
  Equal22/1 -> LiuzgSwitch15/2
  [VINP_PDKeyAreaLockUnlock_enum] -> Equal21/1
  LiuzgSwitch13/1 -> LiuzgSwitch14/3
  Constant43/1 -> Equal20/2
  Equal21/1 -> LiuzgSwitch13/2
  [VINP_PDKeyAreaPS_enum] -> Equal20/1
  Constant47/1 -> Equal22/2
  Equal20/1 -> LiuzgSwitch14/2
  LiuzgSwitch15/1 -> LiuzgSwitch13/3
  Constant45/1 -> Equal21/2
  Constant48/1 -> LiuzgSwitch15/3
  VINP_PDKeyAreaPS_enum/1 -> [VINP_PDKeyAreaPS_enum]
  Hold3/1 -> VPMM_BrkPedalRisingEdge_flg/1  "VPMM_BrkPedalRisingEdge_flg"
  [task_time_s] -> Hold3/1
  Constant41/1 -> Hold3/2
  Detect Increase4/1 -> Hold3/3  "VPMM_BrakePaddleRisingEdge_flg"
  [VPMM_DrivetrainSelect_enum] -> Equal15/1
  LiuzgSwitch10/1 -> LiuzgSwitch11/3
  LiuzgSwitch11/1 -> VPMM_MCUReady_flg/1  "VPMM_MCUReady_flg"
  [VINP_RrMCUReady_flg] -> LiuzgSwitch12/1
  Constant30/1 -> Equal14/2
  Constant28/1 -> LiuzgSwitch12/3
  Equal16/1 -> LiuzgSwitch12/2
  [VPMM_DrivetrainSelect_enum] -> Equal16/1
  AND8/1 -> LiuzgSwitch11/1
  [VINP_FrMCUReady_flg] -> AND8/1
  [VPMM_DrivetrainSelect_enum] -> Equal14/1
  Constant34/1 -> Equal16/2
  LiuzgSwitch12/1 -> LiuzgSwitch10/3
  VINP_RrMCUReady_flg/1 -> [VINP_RrMCUReady_flg]
  Constant32/1 -> Equal15/2
  [VINP_FrMCUReady_flg] -> LiuzgSwitch10/1
  VINP_FrMCUReady_flg/1 -> [VINP_FrMCUReady_flg]
  [VINP_RrMCUReady_flg] -> AND8/2
  Equal14/1 -> LiuzgSwitch11/2
  Equal15/1 -> LiuzgSwitch10/2
  VINP_RrMCUTemp_C/1 -> Terminator5/1
  VINP_RrMCUErr_enum/1 -> Terminator3/1
  VINP_FrMCUTemp_C/1 -> Terminator2/1
  VINP_FrMCUErr_enum/1 -> Terminator/1
  LiuzgSwitch8/1 -> VPMM_MCUDischrgFinished_flg/1  "VPMM_MCUDischrgFinished_flg"
  [VINP_RrDischrgComplete_flg] -> AND4/2
  [VINP_FrDischrgComplete_flg] -> AND4/1
  AND6/1 -> [VINP_FrDischrgComplete_flg]
  AND5/1 -> [VINP_RrDischrgComplete_flg]
  VINP_FrMCUDCBusVolt_V/1 -> [VPMM_FrMCUDCBusVolt_V]
  Constant25/1 -> Equal11/2
  Equal11/1 -> AND6/1
  VINP_FrMCUDischrgSta_flg/1 -> AND6/2
  VINP_RrMCUDischrgSta_flg/1 -> AND5/2
  Equal10/1 -> AND5/1
  Constant24/1 -> Equal10/2
  VINP_RrMCUDCBusVolt_V/1 -> [VPMM_RrMCUDCBusVolt_V]
  [VINP_RrDischrgComplete_flg] -> LiuzgSwitch9/1
  [VPMM_DrivetrainSelect_enum] -> Equal9/1
  Equal9/1 -> LiuzgSwitch9/2
  [VPMM_DrivetrainSelect_enum] -> Equal8/1
  LiuzgSwitch7/1 -> LiuzgSwitch8/3
  Constant19/1 -> Equal4/2
  Equal8/1 -> LiuzgSwitch7/2
  [VPMM_DrivetrainSelect_enum] -> Equal4/1
  Constant23/1 -> Equal9/2
  Equal4/1 -> LiuzgSwitch8/2
  LiuzgSwitch9/1 -> LiuzgSwitch7/3
  Constant21/1 -> Equal8/2
  Constant17/1 -> LiuzgSwitch9/3
  AND4/1 -> LiuzgSwitch8/1
  [VINP_FrDischrgComplete_flg] -> LiuzgSwitch7/1
  [VINP_RrMCUEnaSta_flg] -> AND3/2
  [VINP_FrMCUEnaSta_flg] -> AND3/1
  VINP_RrMCUEnaSta_flg/1 -> [VINP_RrMCUEnaSta_flg]
  VINP_FrMCUEnaSta_flg/1 -> [VINP_FrMCUEnaSta_flg]
  [VINP_FrMCUEnaSta_flg] -> LiuzgSwitch1/1
  AND3/1 -> LiuzgSwitch2/1
  Constant16/1 -> LiuzgSwitch3/3
  Constant6/1 -> Equal2/2
  LiuzgSwitch3/1 -> LiuzgSwitch1/3
  Equal1/1 -> LiuzgSwitch2/2
  Constant8/1 -> Equal3/2
  [VPMM_DrivetrainSelect_enum] -> Equal1/1
  Equal2/1 -> LiuzgSwitch1/2
  Constant4/1 -> Equal1/2
  LiuzgSwitch2/1 -> VPMM_MCUEnable_flg/1  "VPMM_MCUEnable_flg"
  LiuzgSwitch1/1 -> LiuzgSwitch2/3
  [VPMM_DrivetrainSelect_enum] -> Equal2/1
  Equal3/1 -> LiuzgSwitch3/2
  [VPMM_DrivetrainSelect_enum] -> Equal3/1
  [VINP_RrMCUEnaSta_flg] -> LiuzgSwitch3/1
  OR2/1 -> VPMM_AllDoorClosed_flg/1, Detect Increase5/1  "VPMM_AllDoorClosed_flg"
  NOT5/1 -> OR2/4
  NOT4/1 -> OR2/3
  NOT3/1 -> OR2/2
  NOT2/1 -> OR2/1
  AND1/1 -> VPMM_PreChrgChk_flg/1  "VPMM_PreChrgChk_flg"
  VINP_DCDCReady4Pre_flg/1 -> AND1/1
  LiuzgSwitch5/1 -> VPMM_MCUReady4Pre_flg/1, AND1/3  "VPMM_MCUReady4Pre_flg"
  [VINP_FrMCUReady4Pre_flg] -> AND/2
  [VINP_RrMCUReady4Pre_flg] -> AND/1
  VINP_FrMCUReady4Pre_flg/1 -> [VINP_FrMCUReady4Pre_flg]
  VINP_RrMCUReady4Pre_flg/1 -> [VINP_RrMCUReady4Pre_flg]
  [VINP_RrMCUReady4Pre_flg] -> LiuzgSwitch6/1
  [VPMM_DrivetrainSelect_enum] -> Equal6/1
  Equal6/1 -> LiuzgSwitch4/2
  [VINP_FrMCUReady4Pre_flg] -> LiuzgSwitch4/1
  Equal7/1 -> LiuzgSwitch6/2
  LiuzgSwitch4/1 -> LiuzgSwitch5/3
  [VPMM_DrivetrainSelect_enum] -> Equal7/1
  Constant11/1 -> Equal5/2
  Constant15/1 -> Equal7/2
  LiuzgSwitch6/1 -> LiuzgSwitch4/3
  AND/1 -> LiuzgSwitch5/1
  Constant13/1 -> Equal6/2
  Equal5/1 -> LiuzgSwitch5/2
  [VPMM_DrivetrainSelect_enum] -> Equal5/1
  Constant9/1 -> LiuzgSwitch6/3
  VINP_BrakeSWGPIO_flg/1 -> Detect Increase4/1, VPMM_BrkPedalPressed_flg/1
  [VPMM_FlClosed_flg] -> OR1/1
  [VPMM_FrClosed_flg] -> OR1/2
  [VPMM_RlClosed_flg] -> OR1/3
  [VPMM_RrClosed_flg] -> OR1/4
  Hold1/1 -> VPMM_DetectDoorClosed_flg/1  "VPMM_DetectDoorClosed_flg"
  OR1/1 -> Hold1/3
  [task_time_s] -> Hold1/1
  Constant1/1 -> Hold1/2
  Hold/1 -> VPMM_DetectDoorOpened_flg/1  "VPMM_DetectDoorOpened_flg"
  Constant/1 -> Hold/2
  [task_time_s] -> Hold/1
  OR/1 -> Hold/3
  task_time_s/1 -> [task_time_s]
  [VPMM_RrOpened_flg] -> OR/4
  [VPMM_RlOpened_flg] -> OR/3
  [VPMM_FlOpened_flg] -> OR/1
  [VPMM_FrOpened_flg] -> OR/2
  Detect Decrease3/1 -> [VPMM_RrClosed_flg]
  Detect Increase3/1 -> [VPMM_RrOpened_flg]
  Detect Decrease2/1 -> [VPMM_RlClosed_flg]
  Detect Increase2/1 -> [VPMM_RlOpened_flg]
  Detect Decrease1/1 -> [VPMM_FrClosed_flg]
  Detect Increase1/1 -> [VPMM_FrOpened_flg]
  Detect Decrease/1 -> [VPMM_FlClosed_flg]
  Detect Increase/1 -> [VPMM_FlOpened_flg]
  VINP_RLDoorSW_flg/1 -> Detect Increase3/1, Detect Decrease3/1, NOT5/1
  VINP_RRDoorSW_flg/1 -> Detect Increase2/1, Detect Decrease2/1, NOT4/1
  VINP_PsDoorSW_flg/1 -> Detect Increase1/1, Detect Decrease1/1, NOT3/1
  VINP_DrDoorSW_flg/1 -> Detect Increase/1, Detect Decrease/1, NOT2/1
  Constant26/1 -> Switch/2
  VINP_DrivetrainSelect_enum/1 -> [VINP_DrivetrainSelect_enum]
  [VINP_DrivetrainSelect_enum] -> Switch/3
  Constant52/1 -> Switch/1
  Detect Change1/1 -> Logical Operator3/1
  Logical Operator3/1 -> Logical Operator4/2
  Constant54/1 -> Equal17/2
  Logical Operator2/1 -> Logical Operator4/1
  Equal17/1 -> Logical Operator3/2
  Detect Change/1 -> Logical Operator2/1
  Logical Operator4/1 -> VPMM_DetectAntitheftUnlock_flg/1  "VPMM_DetectAntitheftUnlock_flg"
  [VBCM_AntitheftSta_enum] -> Detect Change/1, Equal18/1
  [VBCM_AntitheftSta_enum] -> Detect Change1/1, Equal17/1
  Equal18/1 -> Logical Operator2/2
  Constant53/1 -> Equal18/2
  VBCM_AntitheftSta_enum/1 -> [VBCM_AntitheftSta_enum]
  VINP_DCDCFaultSta_enum/1 -> [VINP_DCDCFaultSta_enum]
  Constant59/1 -> Equal32/2
  Constant58/1 -> Equal33/2
  [VPMM_PDKeySta_enum] -> Equal32/1, Detect Change2/1
  [VPMM_PDKeySta_enum] -> Detect Change3/1, Equal33/1
  Detect Change2/1 -> Logical Operator5/1
  Equal32/1 -> Logical Operator5/2
  Detect Change3/1 -> Logical Operator6/1
  Equal33/1 -> Logical Operator6/2
  Logical Operator5/1 -> Logical Operator7/1
  Logical Operator6/1 -> Logical Operator7/2
  Logical Operator7/1 -> VPMM_DetectPDKeyUnlock_flg/1  "VPMM_DetectPDKeyUnlock_flg"
  [VBCM_AntitheftSta_enum] -> Equal34/1, Detect Change4/1
  Detect Change4/1 -> Logical Operator8/1
  Equal34/1 -> Logical Operator8/2
  Constant60/1 -> Equal34/2
  Constant61/1 -> Equal35/2
  Equal35/1 -> Logical Operator9/2
  Detect Change5/1 -> Logical Operator9/1
  [VBCM_AntitheftSta_enum] -> Detect Change5/1, Equal35/1
  Logical Operator8/1 -> Logical Operator10/1
  Logical Operator9/1 -> Logical Operator10/2
  Logical Operator10/1 -> VPMM_DetectAntitheftLock_flg/1  "VPMM_DetectAntitheftLock_flg"
  [VPMM_PDKeySta_enum] -> Detect Change6/1, Equal36/1
  Constant62/1 -> Equal36/2
  Detect Change6/1 -> Logical Operator11/1
  Equal36/1 -> Logical Operator11/2
  Logical Operator11/1 -> VPMM_DetectPDKeyLock_flg/1  "VPMM_DetectPDKeyLock_flg"
  [task_time_s] -> Hold7/1
  Constant63/1 -> Hold7/2
  Detect Increase8/1 -> Hold7/3
  VINP_IVIPwroffreq_flg/1 -> Detect Increase8/1
  Hold7/1 -> VPMM_DetectIVIPwroffreq_flg/1  "VPMM_DetectIVIPwroffreq_flg"
  Hold8/1 -> VPMM_DetectSchedChg_flg/1  "VPMM_DetectSchedChg_flg"
  Detect Increase9/1 -> Hold8/3
  VINP_SchedChgwake_flg/1 -> Detect Increase9/1
  Constant64/1 -> Hold8/2
  [task_time_s] -> Hold8/1
  [task_time_s] -> Hold9/1
  Constant65/1 -> Hold9/2
  Detect Increase10/1 -> Hold9/3
  VINP_PWCONTINUEUSE_flg/1 -> Detect Increase10/1
  Hold9/1 -> VPMM_DetectPWCONTINUE_flg/1  "VPMM_DetectPWCONTINUE_flg"
  VINP_PDKeyAreaLockUnlock_enum/1 -> [VINP_PDKeyAreaLockUnlock_enum]
  Detect Increase11/1 -> Hold10/3
  Constant66/1 -> Hold10/2
  [task_time_s] -> Hold10/1
  VPMM_HVPwrSta_flg/1 -> Detect Increase11/1
  Hold10/1 -> VPMM_DetectHVPwrSta_flg/1  "VPMM_DetectHVPwrSta_flg"
  VINP_CrashOutputSts_enum/1 -> [VINP_CrashOutputSts_enum]
  [VINP_CrashOutputSts_enum] -> Equal/1
  Constant5/1 -> Equal/2
  Constant67/1 -> Equal37/2
  [VINP_CrashOutputSts_enum] -> Equal37/1
  [VINP_CrashOutputSts_enum] -> Equal38/1
  Constant68/1 -> Equal38/2
  NOT6/1 -> LiuzgSwitch16/1
  Constant70/1 -> LiuzgSwitch27/1
  LiuzgSwitch16/1 -> Timer/2, NOT7/1
  [VINP_BMSWarn6_flg] -> NOT6/1
  Timer/1 -> Equal40/1
  [VPMM_PowerSta_enum] -> Equal41/1
  Constant76/1 -> LiuzgSwitch16/3
  Equal43/1 -> LiuzgSwitch16/2  "VPMM_TMSpdThdSta_flg"
  Constant77/1 -> Equal44/2
  Constant75/1 -> Equal40/2
  Constant69/1 -> Equal43/2
  [task_time_s] -> Timer/3
  [task_time_s] -> Timer1/3
  Equal41/1 -> LiuzgSwitch27/2
  NOT8/1 -> LiuzgSwitch17/3
  NOT7/1 -> Timer/1
  [VPMM_PowerSta_enum] -> Equal44/1
  Constant74/1 -> Timer/4
  Constant72/1 -> Equal41/2
  Equal44/1 -> LiuzgSwitch17/2
  Timer1/1 -> Equal42/1
  Equal42/1 -> NOT11/1
  Logical Operator13/1 -> NOT9/1, Timer1/1
  Equal40/1 -> NOT8/1
  NOT9/1 -> Timer1/2
  [VPMM_TMSpd_rpm] -> Equal43/1
  Constant71/1 -> Timer1/4
  NOT11/1 -> LiuzgSwitch27/3
  Constant79/1 -> Equal42/2
  Constant73/1 -> LiuzgSwitch17/1
  LiuzgSwitch27/1 -> VPMM_SafetyChkHLv_flg/1  "VPMM_SafetyChkHLv_flg"
  LiuzgSwitch17/1 -> VPMM_SafetyChkMLv_flg/1  "VPMM_SafetyChkMLv_flg"
  [VINP_BMSWarn8_flg] -> Logical Operator13/5
  [VINP_BMSWarn7_flg] -> Logical Operator13/4
  Equal38/1 -> Logical Operator13/3
  Equal37/1 -> Logical Operator13/2
  Equal/1 -> Logical Operator13/1
  VINP_HVILSta_flg/1 -> Terminator4/1
  [VINP_BMSWarn6_flg] -> AND7/2
  [VINP_BMSWarn7_flg] -> AND7/3
  [VINP_BMSWarn8_flg] -> AND7/4
  VINP_BMSWarn6_flg/1 -> [VINP_BMSWarn6_flg]
  VINP_BMSWarn8_flg/1 -> [VINP_BMSWarn8_flg]
  VINP_BMSWarn7_flg/1 -> [VINP_BMSWarn7_flg]
  VINP_NewNMSpec_flg/1 -> [VINP_NewNMSpec_flg]
  VINP_VehicleType_enum/1 -> [VINP_VehicleType_enum]
  Constant10/1 -> Equal13/2
  From93/1 -> Equal13/1
  From94/1 -> Logical Operator12/1
  Equal13/1 -> Logical Operator12/2
  Logical Operator12/1 -> LiuzgSwitch19/2
  Gain/1 -> LiuzgSwitch19/1
  LiuzgSwitch19/1 -> VPMM_AuxBatVolt_V_commentout/1, Gain1/1
  VINP_AuxBattVolmV_mV/1 -> [VINP_AuxBattVolmV_mV]
  From95/1 -> Gain/1
  From96/1 -> LiuzgSwitch19/3
  VINP_LVBattDet12V_V/1 -> [VINP_LVBattDet12V_V]
  Equal26/1 -> Logical Operator14/2
  [VINP_NewNMSpec_flg] -> Logical Operator14/1
  [VINP_VehicleType_enum] -> Equal26/1
  Constant12/1 -> Equal26/2
  Logical Operator14/1 -> LiuzgSwitch20/2, LiuzgSwitch21/2
  Gain1/1 -> VPMM_AuxBatVolt_mV_commentout/1
  [VINP_AuxBattVolmV_mV] -> Gain2/1
  [VINP_LVBattDet12V_V] -> LiuzgSwitch20/3
  Gain2/1 -> LiuzgSwitch20/1
  LiuzgSwitch20/1 -> Data Type Conversion3/1
  LiuzgSwitch21/1 -> Data Type Conversion1/1
  Data Type Conversion3/1 -> VPMM_AuxBatVolt_V/1  "VPMM_AuxBatVolt_V"
  Data Type Conversion1/1 -> VPMM_AuxBatVolt_mV/1  "VPMM_AuxBatVolt_mV"
  [VINP_LVBattDet12V_V] -> Gain3/1
  [VINP_AuxBattVolmV_mV] -> LiuzgSwitch21/1
  Gain3/1 -> LiuzgSwitch21/3
  [VINP_DCDCFaultSta_enum] -> Terminator6/1

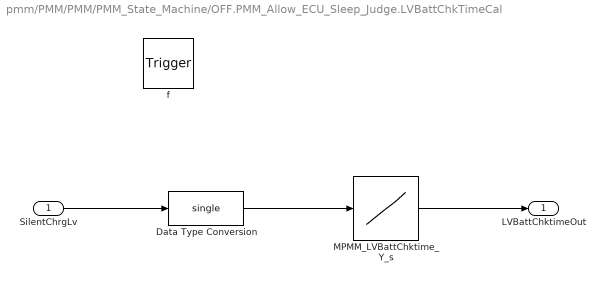
== system pmm/PMM/PMM/PMM_State_Machine/OFF.PMM_Allow_ECU_Sleep_Judge.LVBattChkTimeCal ==
  SilentChrgLv : Inport
  f : TriggerPort  TriggerType=function-call  VariantControl=(inherit)
      settings: CopyFcn=Stateflow.SLINSF.SimulinkMan.removeBlockPreDeleteFcn  PreDeleteFcn=Stateflow.SLINSF.SimulinkMan.unsafePredeleteFcn
  Data Type Conversion : DataTypeConversion  OutDataTypeStr=single
  MPMM_LVBattChktime_Y_s : Lookup_n-D  NumberOfTableDimensions=1  BreakpointsForDimension1=APMM_LVBattChktime_X_enum  Table=MPMM_LVBattChktime_Y_s  ExtrapMethod=Clip  InternalRulePriority=Speed  RndMeth=Simplest  InputSameDT=on
  LVBattChktimeOut : Outport
  wires:
  MPMM_LVBattChktime_Y_s/1 -> LVBattChktimeOut/1
  SilentChrgLv/1 -> Data Type Conversion/1
  Data Type Conversion/1 -> MPMM_LVBattChktime_Y_s/1

== system pmm/PMM/PMM/PMM_State_Machine/OFF.Silent_Charge_Judge.SilentChrgLvCal ==
  LVBatt_mV : Inport
  f : TriggerPort  TriggerType=function-call  VariantControl=(inherit)
      settings: CopyFcn=Stateflow.SLINSF.SimulinkMan.removeBlockPreDeleteFcn  PreDeleteFcn=Stateflow.SLINSF.SimulinkMan.unsafePredeleteFcn
  MPMM_LVChrgLv_Y_Lv : Lookup_n-D  NumberOfTableDimensions=1  BreakpointsForDimension1=APMM_LVChrgLv_X_mV  Table=MPMM_LVChrgLv_Y_Lv  ExtrapMethod=Clip  InternalRulePriority=Speed  RndMeth=Simplest  InputSameDT=on
  SilentChrgLv : Outport
  wires:
  LVBatt_mV/1 -> MPMM_LVChrgLv_Y_Lv/1
  MPMM_LVChrgLv_Y_Lv/1 -> SilentChrgLv/1  "VPMM_LVChrgLvOut_enum"

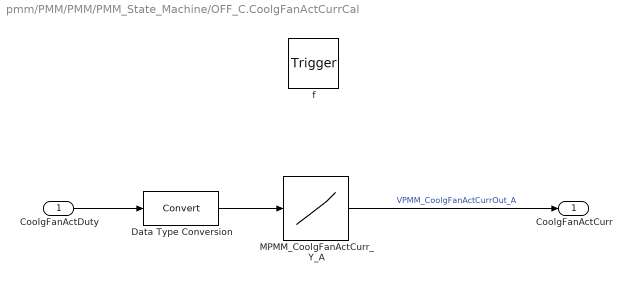
== system pmm/PMM/PMM/PMM_State_Machine/OFF_C.CoolgFanActCurrCal ==
  CoolgFanActDuty : Inport
  f : TriggerPort  TriggerType=function-call  VariantControl=(inherit)
      settings: CopyFcn=Stateflow.SLINSF.SimulinkMan.removeBlockPreDeleteFcn  PreDeleteFcn=Stateflow.SLINSF.SimulinkMan.unsafePredeleteFcn
  Data Type Conversion : DataTypeConversion
  MPMM_CoolgFanActCurr_Y_A : Lookup_n-D  NumberOfTableDimensions=1  BreakpointsForDimension1=APMM_CoolgFanActCurr_X_pct  Table=MPMM_CoolgFanActCurr_Y_A  ExtrapMethod=Clip  InternalRulePriority=Speed  RndMeth=Simplest  InputSameDT=on
  CoolgFanActCurr : Outport
  wires:
  MPMM_CoolgFanActCurr_Y_A/1 -> CoolgFanActCurr/1  "VPMM_CoolgFanActCurrOut_A"
  CoolgFanActDuty/1 -> Data Type Conversion/1
  Data Type Conversion/1 -> MPMM_CoolgFanActCurr_Y_A/1

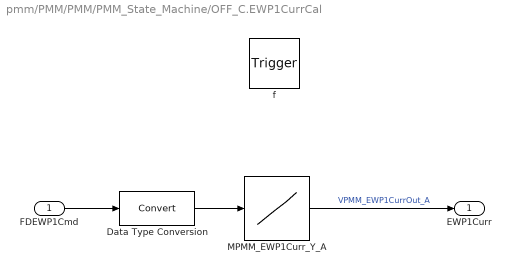
== system pmm/PMM/PMM/PMM_State_Machine/OFF_C.EWP1CurrCal ==
  FDEWP1Cmd : Inport
  f : TriggerPort  TriggerType=function-call  VariantControl=(inherit)
      settings: CopyFcn=Stateflow.SLINSF.SimulinkMan.removeBlockPreDeleteFcn  PreDeleteFcn=Stateflow.SLINSF.SimulinkMan.unsafePredeleteFcn
  Data Type Conversion : DataTypeConversion
  MPMM_EWP1Curr_Y_A : Lookup_n-D  NumberOfTableDimensions=1  BreakpointsForDimension1=APMM_EWP1Curr_X_c  Table=MPMM_EWP1Curr_Y_A  ExtrapMethod=Clip  InternalRulePriority=Speed  RndMeth=Simplest  InputSameDT=on
  EWP1Curr : Outport
  wires:
  MPMM_EWP1Curr_Y_A/1 -> EWP1Curr/1  "VPMM_EWP1CurrOut_A"
  FDEWP1Cmd/1 -> Data Type Conversion/1
  Data Type Conversion/1 -> MPMM_EWP1Curr_Y_A/1

== system pmm/PMM/PMM/PMM_State_Machine/OFF_C.EWP3CurrCal ==
  FDEWP3Cmd : Inport
  f : TriggerPort  TriggerType=function-call  VariantControl=(inherit)
      settings: CopyFcn=Stateflow.SLINSF.SimulinkMan.removeBlockPreDeleteFcn  PreDeleteFcn=Stateflow.SLINSF.SimulinkMan.unsafePredeleteFcn
  Data Type Conversion : DataTypeConversion
  MPMM_EWP3Curr_Y_A : Lookup_n-D  NumberOfTableDimensions=1  BreakpointsForDimension1=APMM_EWP3Curr_X_c  Table=MPMM_EWP3Curr_Y_A  ExtrapMethod=Clip  InternalRulePriority=Speed  RndMeth=Simplest  InputSameDT=on
  EWP3Curr : Outport
  wires:
  MPMM_EWP3Curr_Y_A/1 -> EWP3Curr/1  "VPMM_EWP3CurrOut_A"
  FDEWP3Cmd/1 -> Data Type Conversion/1
  Data Type Conversion/1 -> MPMM_EWP3Curr_Y_A/1
